simulink model "frequency_count_v2"  (Simulink 10.1)
settings: Solver=ode45  StartTime=0.0  StopTime=2.5  FixedStep=5e-6  RelTol=1e-4  EnableMultiTasking=on
libraries: simulink x1
settings Model: Creator=mf  LastModifiedBy=Robin Vogt  ExtModeAutoUpdateStatusClock=off
settings DataIOCC: LimitDataPoints=on  SignalLoggingSaveFormat=ModelDataLogs  SignalLoggingName=sigsOut
settings OptimizationCC: BooleanDataType=off  ExpressionDepthLimit=2147483647
settings DebuggingCC: SaveWithParameterizedLinksMsg=none  SignalResolutionControl=TryResolveAllWithWarning  MultiTaskDSMMsg=warning  MultiTaskCondExecSysMsg=none  StateNameClashWarn=warning
settings HardwareCC: TargetUnknown=on
settings SFSimCC: SimParseCustomCode=off

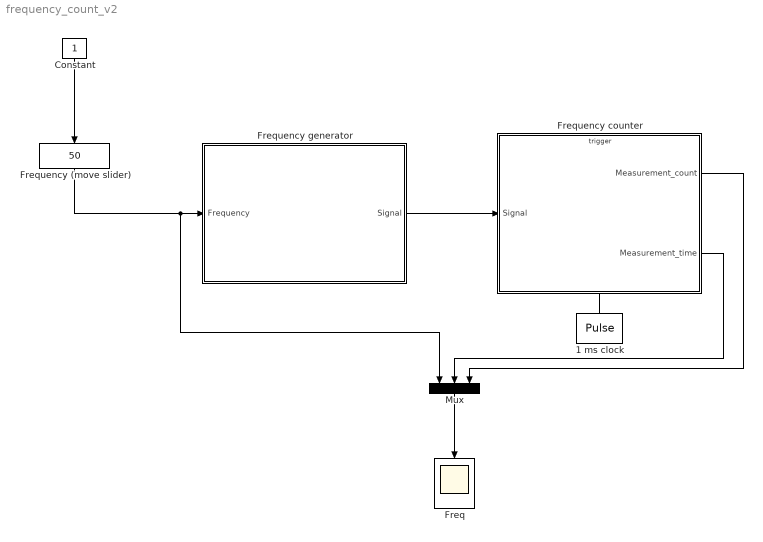
== system frequency_count_v2 ==
  1 ms clock : DiscretePulseGenerator  PulseType=Time based  Period=1e-3  PulseWidth=50
  Constant : Constant
  Freq : Scope
  Frequency (move slider) : simulink/Math Operations/Slider Gain  gain=50  low=1  high=500
  Frequency counter : Stateflow chart  TreatAsAtomicUnit=on
  Frequency generator : Subsystem
  Mux : Mux  Inputs=3
  wires:
  Frequency generator/1(Signal) -> Frequency counter/1(Signal)
  Constant/1 -> Frequency (move slider)/1
  1 ms clock/1 -> Frequency counter/Trigger
  Mux/1 -> Freq/1
  Frequency (move slider)/1 -> Frequency generator/1(Frequency), Mux/1
  Frequency counter/1(Measurement_count) -> Mux/3
  Frequency counter/2(Measurement_time) -> Mux/2

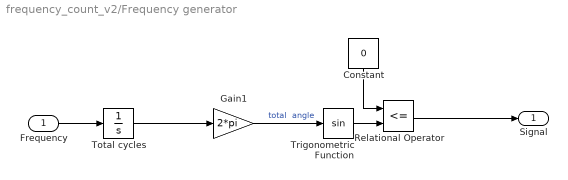
== system frequency_count_v2/Frequency generator ==
  Frequency : Inport
  Constant : Constant  Value=0
  Gain1 : Gain  Gain=2*pi  SaturateOnIntegerOverflow=on  OutDataTypeStr=Inherit: Same as input  ParamDataTypeStr=Inherit: Same as input
  Relational Operator : RelationalOperator  Operator=<=  OutDataTypeStr=boolean  RndMeth=Nearest
  Total cycles : Integrator
  Trigonometric Function : Trigonometry
  Signal : Outport
  wires:
  Frequency/1 -> Total cycles/1
  Trigonometric Function/1 -> Relational Operator/2
  Constant/1 -> Relational Operator/1
  Relational Operator/1 -> Signal/1
  Total cycles/1 -> Gain1/1
  Gain1/1 -> Trigonometric Function/1  "total  angle"

== stateflow chart Frequency counter ==
  settings: executeAtInitialization=1
  state FrequencyCounter
    state Measuring_Count [parallel]
      settings: executionOrder=2
      state Counter [parallel]
        settings: executionOrder=2
        state Signal_Counter
        (default) -> Signal_Counter
        Signal_Counter -> Signal_Counter : [hasChanged(Signal)]/{signal_count ++;}
      state Timer [parallel]
        settings: executionOrder=1
        state Clk_Counter/
          en:
          clk_count_c = 0;
          du:
          clk_count_c ++;
        (default) -> Clk_Counter
        Clk_Counter -> Clk_Counter : [clk_count_c == time_interval_multiplier]/{
            | Measurement_count = (500*signal_count)/time_interval_multiplier;
            | signal_count = 0;
            | clk_count_c = 0;}
    state Measuring_Time [parallel]
      settings: executionOrder=1
      state Signal_false
      state Signal_true
      (default) -> Signal_true
      Signal_false -> Signal_false [order 2] : {clk_count_t ++;}
      Signal_true -> Signal_false [order 1] : [~Signal]/{clk_count_t ++;}
      Signal_true -> Signal_true [order 2] : {clk_count_t ++;}
      Signal_false -> Signal_true [order 1] : [Signal]/{
          | Measurement_time = uint64(1000)/clk_count_t;
          | clk_count_t = 1;
          | }
  data: Signal input boolean; Measurement_count output double =0; signal_count local uint64 =uint64(0); Measurement_time output double =0; clk_count_c local uint64 =uint64(0); clk_count_t local uint64 =uint64(0); time_interval_multiplier constant uint8 =uint8(100)
  events: clk input RISING_EDGE_EVENT
